simulink model "Module 4"  (R2021b)
settings: Solver=FixedStepAuto  StartTime=0.0  StopTime=10.0  RelTol=1e-3
libraries: simulink x2
settings Model: Creator=Lenovo  LastModifiedBy=Lenovo

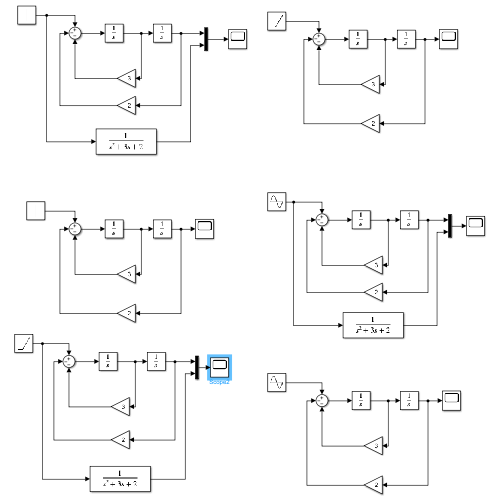
[thumbnail: Simulink's stored preview of the top-level diagram]
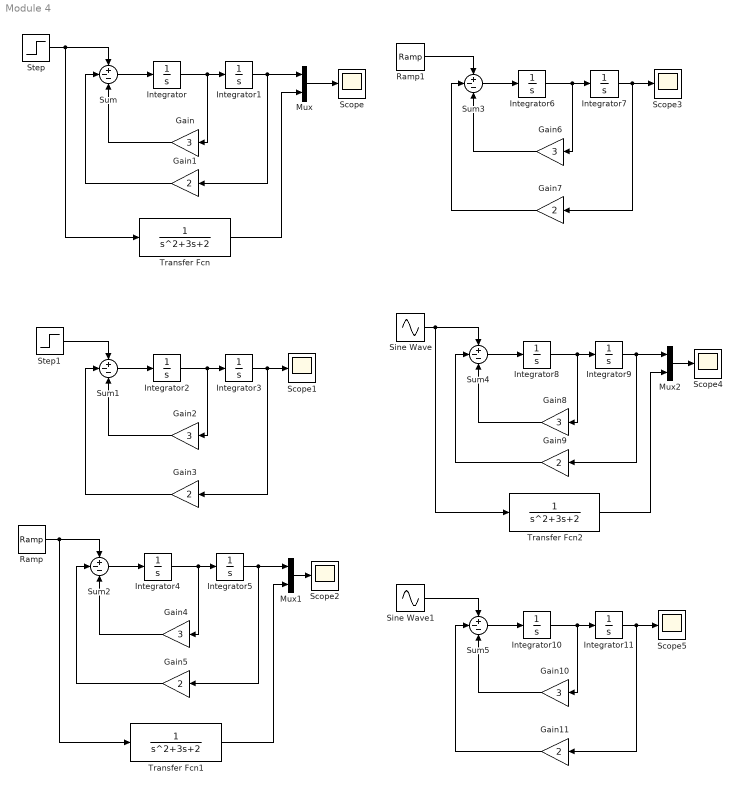
== system Module 4 ==
  Gain{,2,4,6,8,10} (6 alike) : Gain  Gain=3
  Gain{1,3,5,7,9,11} (6 alike) : Gain  Gain=2
  Integrator{,1..2,4..6,8..10} (9 alike) : Integrator
  Integrator11 : Integrator  InitialCondition=-1
  Integrator3 : Integrator  InitialCondition=0.1
  Integrator7 : Integrator  InitialCondition=0.1
  Mux : Mux  Inputs=2
  Mux1 : Mux  Inputs=2
  Mux2 : Mux  Inputs=2
  Ramp : simulink/Sources/Ramp  slope=1  start=0  InitialOutput=1
  Ramp1 : simulink/Sources/Ramp  slope=1  start=0  InitialOutput=1
  Scope{,1..5} (6 alike) : Scope
  Sine Wave : Sin  Amplitude=3  Frequency=6*pi  SampleTime=0
  Sine Wave1 : Sin  Amplitude=3  Frequency=6*pi  SampleTime=0
  Step : Step  Time=0  SampleTime=0
  Step1 : Step  Time=0  SampleTime=0
  Sum{,1..5} (6 alike) : Sum  Inputs=+--
  Transfer Fcn : TransferFcn  Denominator=[1 3 2]
  Transfer Fcn1 : TransferFcn  Denominator=[1 3 2]
  Transfer Fcn2 : TransferFcn  Denominator=[1 3 2]
  wires:
  Sum/1 -> Integrator/1
  Integrator/1 -> Gain/1, Integrator1/1
  Integrator1/1 -> Mux/1, Gain1/1
  Gain/1 -> Sum/3
  Gain1/1 -> Sum/2
  Step/1 -> Transfer Fcn/1, Sum/1
  Integrator2/1 -> Gain2/1, Integrator3/1
  Sum1/1 -> Integrator2/1
  Gain3/1 -> Sum1/2
  Gain2/1 -> Sum1/3
  Integrator3/1 -> Gain3/1, Scope1/1
  Step1/1 -> Sum1/1
  Ramp/1 -> Transfer Fcn1/1, Sum2/1
  Integrator5/1 -> Mux1/1, Gain5/1
  Sum2/1 -> Integrator4/1
  Gain4/1 -> Sum2/3
  Integrator4/1 -> Gain4/1, Integrator5/1
  Gain5/1 -> Sum2/2
  Gain7/1 -> Sum3/2
  Gain6/1 -> Sum3/3
  Sum3/1 -> Integrator6/1
  Integrator7/1 -> Gain7/1, Scope3/1
  Ramp1/1 -> Sum3/1
  Integrator6/1 -> Gain6/1, Integrator7/1
  Gain9/1 -> Sum4/2
  Sum4/1 -> Integrator8/1
  Integrator8/1 -> Gain8/1, Integrator9/1
  Gain8/1 -> Sum4/3
  Sine Wave/1 -> Transfer Fcn2/1, Sum4/1
  Integrator9/1 -> Mux2/1, Gain9/1
  Sine Wave1/1 -> Sum5/1
  Gain10/1 -> Sum5/3
  Sum5/1 -> Integrator10/1
  Integrator10/1 -> Gain10/1, Integrator11/1
  Integrator11/1 -> Gain11/1, Scope5/1
  Gain11/1 -> Sum5/2
  Mux1/1 -> Scope2/1
  Transfer Fcn1/1 -> Mux1/2
  Mux2/1 -> Scope4/1
  Transfer Fcn2/1 -> Mux2/2
  Transfer Fcn/1 -> Mux/2
  Mux/1 -> Scope/1
